simulink model "as1_3"  (R2023b)
settings: Solver=VariableStepAuto  StartTime=0.0  StopTime=10.0  RelTol=1e-3
values from neighbouring files (symbols this model uses):
  b = 0.1    [main.m]
  g = 9.8    [main.m]
  Kd = KdArray(j)    [main.m]
  Kp = KpArray(i)    [main.m]
  l = 1    [main.m]
  m = 1    [main.m]
  thetaDotNoiseGain = 3    [main.m]
  thetaNoiseGain = 3    [main.m]
  x1 = pi    (= 3.14159265359)    [main.m]
  x2 = 0    [main.m]
settings Model: Creator=Shadow  LastModifiedBy=Shadow

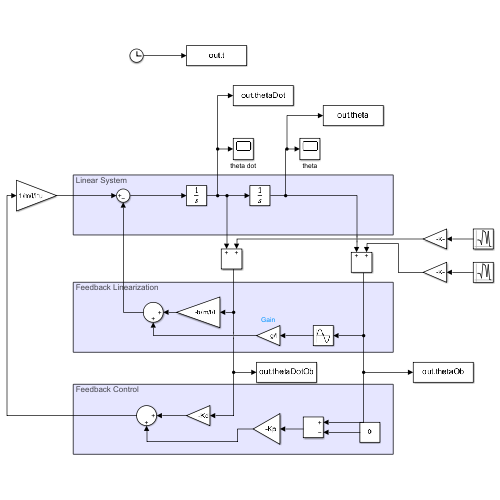
[thumbnail: Simulink's stored preview of the top-level diagram]
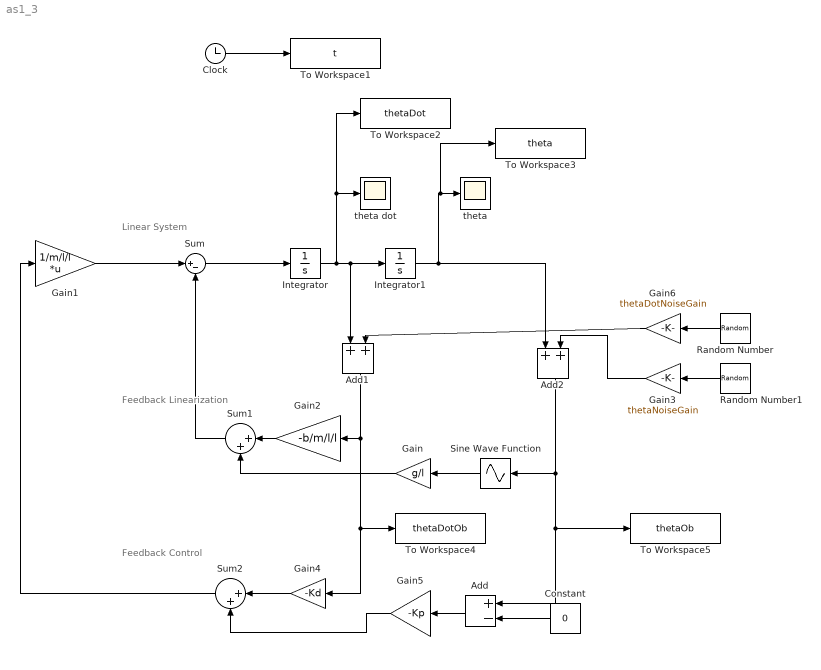
== system as1_3 ==
  note: Feedback Linearization
  note: Linear System
  note: Feedback Control
  Add : Sum  Inputs=+-
  Add1 : Sum
  Add2 : Sum
  Clock : Clock
  Constant : Constant  Value=0
  Gain : Gain  Gain=g/l
  Gain1 : Gain  Gain=1/m/l/l  Multiplication=Matrix(K*u)
  Gain2 : Gain  Gain=-b/m/l/l
  Gain3 : Gain  Gain=thetaNoiseGain
  Gain4 : Gain  Gain=-Kd
  Gain5 : Gain  Gain=-Kp
  Gain6 : Gain  Gain=thetaDotNoiseGain
  Integrator : Integrator  InitialCondition=x2
  Integrator1 : Integrator  InitialCondition=x1
  Random Number : RandomNumber  SampleTime=0.001
  Random Number1 : RandomNumber  SampleTime=0.001
  Sine Wave Function : Sin  TimeSource=Use external signal  SampleTime=0
  Sum : Sum  Inputs=|+-
  Sum1 : Sum  Inputs=|++
  Sum2 : Sum  Inputs=|++
  To Workspace1 : ToWorkspace  VariableName=t  SampleTime=0.01
      settings: Save2DSignal=2-D array (concatenate along first dimension)
  To Workspace2 : ToWorkspace  VariableName=thetaDot  SampleTime=0.01
      settings: Save2DSignal=2-D array (concatenate along first dimension)
  To Workspace3 : ToWorkspace  VariableName=theta  SampleTime=0.01
      settings: Save2DSignal=2-D array (concatenate along first dimension)
  To Workspace4 : ToWorkspace  VariableName=thetaDotOb  SampleTime=0.01
      settings: Save2DSignal=2-D array (concatenate along first dimension)
  To Workspace5 : ToWorkspace  VariableName=thetaOb  SampleTime=0.01
      settings: Save2DSignal=2-D array (concatenate along first dimension)
  theta : Scope
  theta dot : Scope
  wires:
  Sum/1 -> Integrator/1
  Integrator/1 -> Add1/1, Integrator1/1, To Workspace2/1, theta dot/1
  Clock/1 -> To Workspace1/1
  Integrator1/1 -> Add2/1, To Workspace3/1, theta/1
  Sine Wave Function/1 -> Gain/1
  Gain/1 -> Sum1/2
  Gain2/1 -> Sum1/1
  Sum1/1 -> Sum/2
  Gain1/1 -> Sum/1
  Constant/1 -> Add/2
  Add/1 -> Gain5/1
  Gain5/1 -> Sum2/2
  Gain4/1 -> Sum2/1
  Sum2/1 -> Gain1/1
  Random Number/1 -> Gain6/1
  Add1/1 -> To Workspace4/1, Gain4/1, Gain2/1
  Add2/1 -> To Workspace5/1, Add/1, Sine Wave Function/1
  Gain6/1 -> Add1/2
  Gain3/1 -> Add2/2
  Random Number1/1 -> Gain3/1
